simulink model "final_project"  (R2019b)
settings: Solver=VariableStepAuto  StartTime=0.0  StopTime=10.0  RelTol=1e-3
libraries: robotmobilelib x2, simulink x1
settings Model: Creator=Mertcan  LastModifiedBy=Mertcan

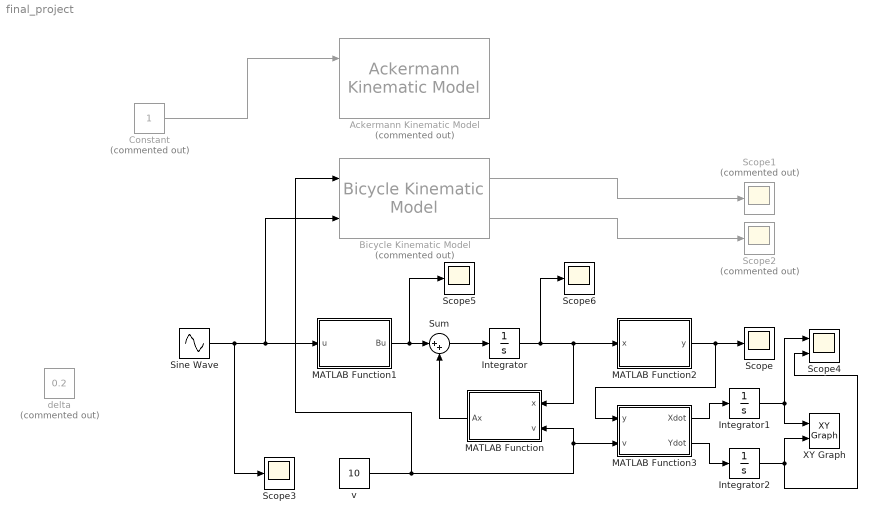
== system final_project ==
  Ackermann Kinematic Model : robotmobilelib/Ackermann Kinematic Model  Commented=on  WheelBase=1  VehicleSpeedRange=[-inf inf]  MaxSteeringAngle=pi/4  InitialState=[0; 0; 0; 0]  SimulateUsing=Interpreted execution
      settings: SourceProductName=Robotics System Toolbox  SourceProductBaseCode=RO
  Bicycle Kinematic Model : robotmobilelib/Bicycle Kinematic Model  Commented=on  VehicleInputs=Vehicle Speed & Steering Angle  WheelBase=1  VehicleSpeedRange=[-inf inf]  MaxSteeringAngle=pi/4  InitialState=[0; 0; 0]  SimulateUsing=Interpreted execution
      settings: SourceProductName=Robotics System Toolbox  SourceProductBaseCode=RO
  Constant : Constant  Commented=on
  Integrator : Integrator
  Integrator1 : Integrator
  Integrator2 : Integrator
  MATLAB Function : MATLAB Function  TreatAsAtomicUnit=on
  MATLAB Function1 : MATLAB Function  TreatAsAtomicUnit=on
  MATLAB Function2 : MATLAB Function  TreatAsAtomicUnit=on
  MATLAB Function3 : MATLAB Function  TreatAsAtomicUnit=on
  Scope{,3,5..6} (4 alike) : Scope
  Scope1 : Scope  Commented=on
  Scope2 : Scope  Commented=on
  Scope4 : Scope  NumInputPorts=2
  Sine Wave : Sin  Amplitude=0.07  SampleTime=0
  Sum : Sum  Inputs=|++
  XY Graph : simulink/Sinks/XY Graph  xmin=-1  xmax=100  ymin=-10  ymax=30  st=-1
  delta : Constant  Commented=on  Value=0.2
  v : Constant  Value=10
  wires:
  Constant/1 -> Ackermann Kinematic Model/1
  Sum/1 -> Integrator/1
  MATLAB Function/1(Ax) -> Sum/2
  MATLAB Function1/1(Bu) -> Scope5/1, Sum/1
  Integrator/1 -> Scope6/1, MATLAB Function2/1(x), MATLAB Function/1(x)
  Sine Wave/1 -> Scope3/1, Bicycle Kinematic Model/2, MATLAB Function1/1(u)
  v/1 -> Bicycle Kinematic Model/1, MATLAB Function3/2(v), MATLAB Function/2(v)
  MATLAB Function2/1(y) -> MATLAB Function3/1(y), Scope/1
  Bicycle Kinematic Model/1 -> Scope1/1
  Bicycle Kinematic Model/2 -> Scope2/1
  MATLAB Function3/1(Xdot) -> Integrator1/1
  Integrator1/1 -> Scope4/1, XY Graph/1
  Integrator2/1 -> XY Graph/2, Scope4/2
  MATLAB Function3/2(Ydot) -> Integrator2/1

== matlab function final_project/MATLAB Function1 ==
  data: u input; Bu output
function Bu = Bmat(u)

m = 1350; % kg
lf = 1.016; % m
Iz = 4000; % kg.m^2
Cf = 87594; % N/rad

B = [0;Cf/m;0;(Cf*lf)/Iz];

Bu = B*u;

== matlab function final_project/MATLAB Function ==
  data: x input; Ax output; v input
function Ax = Amat(x,v)

m = 1350; % kg
lf = 1.016; % m
lr = 1.562; % m
Iz = 4000; % kg.m^2
Cf = 87594; % N/rad
Cr = 87594; % N/rad

a22 = -(Cf+Cr)/(m*v);
a24 = (Cr*lr-Cf*lf)/(m*v)-v;
a42 = (Cr*lr-Cf*lf)/(Iz*v);
a44 = (-Cr*lr^2-Cf*lf^2)/(Iz*v);

A = [0, 1, 0, 0
    0, a22, 0, a24
    0, 0, 0, 1
    0, a42, 0, a44];

Ax = A*x;

== matlab function final_project/MATLAB Function2 ==
  data: x input; y output
function y = Cmat(x)

C = [1, 0, 0, 0
    0, 0, 1, 0];

y = C*x;

== matlab function final_project/MATLAB Function3 ==
  data: y input; Xdot output; v input; Ydot output
function [Xdot, Ydot] = CmatXY(y,v)

ydot = y(1);
phi = y(2);

Ydot = sin(phi)*v+cos(phi)*ydot;
Xdot = cos(phi)*v-sin(phi)*ydot;
